simulink model "Assignment1"  (R2020a)
settings: Solver=FixedStepAuto  StartTime=0.0  StopTime=10.0  FixedStep=1e-3  RelTol=1e-3  EnableMultiTasking=on
undefined symbols (not defined in the file): D0, D1, D10, D11, D12, D13, D2, D3, D4, D5, D6, D7, D8, D9, PTA0, PTA1, PTA2, PTB23, PTB9, PTC16, PTC17, PTC2, PTC3, PTC4, PTD0, PTD1, PTD2, PTD3
libraries: frdmk64flib x14
settings Model: ExtModeTrigDuration=5  Creator=iceca  LastModifiedBy=iceca
settings OptimizationCC: EnhancedBackFolding=on  PassReuseOutputArgsAs=Individual arguments  ZeroExternalMemoryAtStartup=off  ZeroInternalMemoryAtStartup=off  MaxStackSize=64  OptimizeBlockOrder=speed  DifferentSizesBufferReuse=on  OptimizationCustomize=off  EfficientTunableParamExpr=on
settings DebuggingCC: ParameterTunabilityLossMsg=error
settings HardwareCC: ProdBitPerPointer=32  ProdBitPerSizeT=32  ProdBitPerPtrDiffT=32  ProdLargestAtomicInteger=Long  ProdLargestAtomicFloat=Double  ProdWordSize=32  ProdHWDeviceType=ARM Compatible->ARM Cortex
settings SFSimCC: MATLABDynamicMemAlloc=off
settings RTWCC: SystemTargetFile=ert.tlc  HardwareBoard=NXP FRDM-K64F  TemplateMakefile=ert_default_tmf  Toolchain=GNU Tools for ARM Embedded Processors
settings CodeAppCC: ForceParamTrailComments=on  IgnoreCustomStorageClasses=off  OperatorAnnotations=on  SimulinkDataObjDesc=on  SFDataObjDesc=on  InsertBlockDesc=on

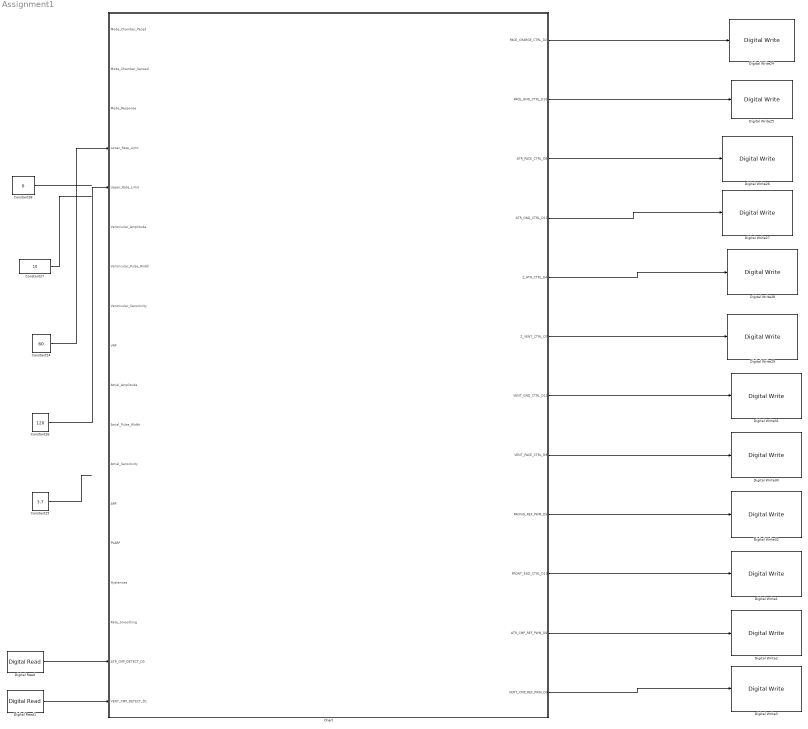
== system Assignment1 ==
  Chart : Stateflow chart  TreatAsAtomicUnit=on
  Constant24 : Constant  Value=60
  Constant25 : Constant  Value=3.7
  Constant26 : Constant  Value=120
  Constant27 : Constant  Value=10
  Constant28 : Constant  Value=0
  Digital Read : frdmk64flib/Digital Read  Whichpin=PTC16 (D0)  SampleTime=-1
  Digital Read1 : frdmk64flib/Digital Read  Whichpin=PTC17 (D1)  SampleTime=-1
  Digital Write1 : frdmk64flib/Digital Write  Whichpin=PTD1 (D13)
  Digital Write2 : frdmk64flib/Digital Write  Whichpin=PTC2 (D6)
  Digital Write24 : frdmk64flib/Digital Write  Whichpin=PTB9 (D2)
  Digital Write25 : frdmk64flib/Digital Write  Whichpin=PTD0 (D10)
  Digital Write26 : frdmk64flib/Digital Write  Whichpin=PTA0 (D8)
  Digital Write27 : frdmk64flib/Digital Write  Whichpin=PTD2 (D11)
  Digital Write28 : frdmk64flib/Digital Write  Whichpin=PTB23 (D4)
  Digital Write29 : frdmk64flib/Digital Write  Whichpin=PTC3 (D7)
  Digital Write3 : frdmk64flib/Digital Write  Whichpin=PTA1 (D3)
  Digital Write30 : frdmk64flib/Digital Write  Whichpin=PTC4 (D9)
  Digital Write31 : frdmk64flib/Digital Write  Whichpin=PTD3 (D12)
  Digital Write32 : frdmk64flib/Digital Write  Whichpin=PTA2 (D5)
  wires:
  Constant27/1 -> ?
  Chart/9(PACING_REF_PWM_D5) -> Digital Write32/1
  Constant24/1 -> Chart/4(Lower_Rate_Limit)
  Chart/5(Z_ATR_CTRL_D4) -> Digital Write28/1
  Chart/7(VENT_GND_CTRL_D12) -> Digital Write31/1
  Constant28/1 -> ?
  Chart/8(VENT_PACE_CTRL_D9) -> Digital Write30/1
  Chart/2(PACE_GND_CTRL_D10) -> Digital Write25/1
  Constant25/1 -> ?
  Constant26/1 -> Chart/5(Upper_Rate_Limit)
  Chart/3(ATR_PACE_CTRL_D8) -> Digital Write26/1
  Chart/4(ATR_GND_CTRL_D11) -> Digital Write27/1
  Chart/6(Z_VENT_CTRL_D7) -> Digital Write29/1
  Chart/1(PACE_CHARGE_CTRL_D2) -> Digital Write24/1
  Chart/10(FRONT_END_CTRL_D13) -> Digital Write1/1
  Chart/11(ATR_CMP_REF_PWM_D6) -> Digital Write2/1
  Chart/12(VENT_CMP_REF_PWM_D3) -> Digital Write3/1
  Digital Read1/1 -> Chart/18(VENT_CMP_DETECT_D1)
  Digital Read/1 -> Chart/17(ATR_CMP_DETECT_D0)

== stateflow chart Assignment1/Chart ==
  state Discharching_C21_and_Charging_C23
    entry:
    %Charging C22
    ATR_PACE_CTRL_D8   = LOW;
    VENT_PACE_CTRL_D9 = LOW;
    if Mode_Chamber_Paced==1
    PACING_REF_PWM_D5 = Atrial_Amplitude*20;
    else
    PACING_REF_PWM_D5 = Ventricular_Amplitude*20;
    end
    PACE_CHARGE_CTRL_D2 = HIGH;
    %Calculating Rate and Period
    avgRate = (Lower_Rate_Limit+Upper_Rate_Limit)/2;
    Period = 60000/avgRate;
    %Discharging C21
    PACE_GND_CTRL_D10=HIGH;
    VENT_PACE_CTRL_D9=LOW;
    Z_ATR_CTRL_D4 = LOW;
    Z_VENT_CTRL_D7 = LOW;
    ATR_PACE_CTRL_D8 = LOW;
  state Ventricular_Discharge_Charge
    entry:
    ATR_GND_CTRL_D11 = LOW;
    VENT_GND_CTRL_D12 = HIGH;
  state Atrial_Discharge_Charge
    entry:
    ATR_GND_CTRL_D11 = HIGH;
    VENT_GND_CTRL_D12= LOW;
  state Discharge_Charge_Complete
  state Ventricular_Sensing
    during:
    VENT_CMP_REF_PWM_D3 = 20*Ventricular_Sensitivity;
  state Sensing
    entry:
    FRONT_END_CTRL_D13 = HIGH;
  state Natural_Activity_Detected
  state Atrial_Sensing
    during:
    ATR_CMP_REF_PWM_D6= 20*Atrial_Sensitivity;
  state No_Natural_Activity_Sensed
  state Pacing
    entry:
    PACE_CHARGE_CTRL_D2 = 0;
    PACE_GND_CTRL_D10 = 1;
    ATR_PACE_CTRL_D8 = 0;
    ATR_GND_CTRL_D11 =0;
    Z_ATR_CTRL_D4 = 0;
    Z_VENT_CTRL_D7 = 0;
    VENT_GND_CTRL_D12 = 0;
  state Ventricular_Pacing
    entry:
    ATR_PACE_CTRL_D8 =0;
    VENT_PACE_CTRL_D9 =1;
  state Atrial_Pacing
    during:
    VENT_PACE_CTRL_D9 =0;
    ATR_PACE_CTRL_D8 =1;
  state Pacing_Complete
  Pacing_Complete -> Discharching_C21_and_Charging_C23
  Natural_Activity_Detected -> Discharching_C21_and_Charging_C23
  (default) -> Discharching_C21_and_Charging_C23
  Discharching_C21_and_Charging_C23 -> Atrial_Discharge_Charge [order 1] : [Mode_Chamber_Paced==1]
  Discharching_C21_and_Charging_C23 -> Ventricular_Discharge_Charge [order 2] : [Mode_Chamber_Paced==2]
  Ventricular_Discharge_Charge -> Discharge_Charge_Complete
  Atrial_Discharge_Charge -> Discharge_Charge_Complete
  Discharge_Charge_Complete -> No_Natural_Activity_Sensed [order 2] : [Mode_Chamber_Sensed==0]
  Discharge_Charge_Complete -> Sensing [order 1] : [Mode_Chamber_Sensed~=0]
  Ventricular_Sensing -> Natural_Activity_Detected [order 1] : [Mode_Response==1 &&  VENT_CMP_DETECT_D1==1 && after(VRP, msec)]
  Sensing -> Ventricular_Sensing [order 1] : [Mode_Chamber_Sensed==2]
  Sensing -> Atrial_Sensing [order 2] : [Mode_Chamber_Sensed==1]
  Ventricular_Sensing -> No_Natural_Activity_Sensed [order 2] : [after(Period-Ventricular_Pulse_Width,msec)]
  Atrial_Sensing -> Natural_Activity_Detected [order 1] : [Mode_Response==1 &&  ATR_CMP_DETECT_D0==1 && after(ARP, msec)]
  Atrial_Sensing -> No_Natural_Activity_Sensed [order 2] : [after(Period-Atrial_Pulse_Width,msec)]
  No_Natural_Activity_Sensed -> Pacing
  Pacing -> Atrial_Pacing [order 2] : [Mode_Chamber_Paced==1]
  Pacing -> Ventricular_Pacing [order 1] : [Mode_Chamber_Paced==2]
  Ventricular_Pacing -> Pacing_Complete : [after(Ventricular_Pulse_Width,msec)]
  Atrial_Pacing -> Pacing_Complete : [after(Atrial_Pulse_Width,msec)]
  data: Mode_Chamber_Paced input; Mode_Chamber_Sensed input; Mode_Response input; PACE_CHARGE_CTRL_D2 output; PACE_GND_CTRL_D10 output; ATR_PACE_CTRL_D8 output; ATR_GND_CTRL_D11 output; Z_ATR_CTRL_D4 output; Z_VENT_CTRL_D7 output; VENT_GND_CTRL_D12 output; VENT_PACE_CTRL_D9 output; PACING_REF_PWM_D5 output; avgRate local double; Lower_Rate_Limit input; Upper_Rate_Limit input; HIGH local boolean =true; LOW local boolean =false; Ventricular_Amplitude input; Ventricular_Pulse_Width input; Ventricular_Sensitivity input; VRP input; Atrial_Amplitude input; Atrial_Pulse_Width input; Atrial_Sensitivity input; ARP input; PVARP input; Hysterises input; Rate_Smoothing input; Period local; FRONT_END_CTRL_D13 output; ATR_CMP_REF_PWM_D6 output; VENT_CMP_REF_PWM_D3 output; ATR_CMP_DETECT_D0 input; VENT_CMP_DETECT_D1 input
